simulink model "sing_phase_inv"  (R2020b)
settings: Solver=VariableStepAuto  StartTime=0.0  StopTime=0.3  RelTol=1e-3
libraries: spsMosfetLib x4, spsCurrentMeasurementLib x2, simulink x1, spsDCVoltageSourceLib x1, spsSeriesRLCBranchLib x1, spsVoltageMeasurementLib x1, spspowerguiLib x1
settings Model: Creator=win10  LastModifiedBy=mansi
settings DataIOCC: ReturnWorkspaceOutputs=off

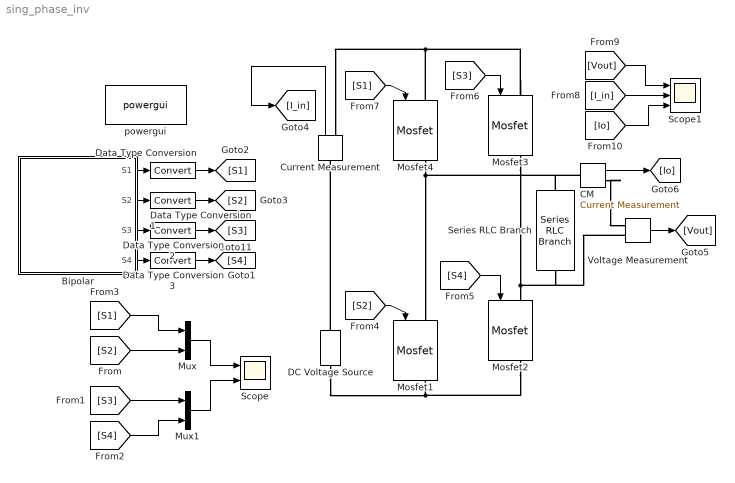
== system sing_phase_inv ==
  Bipolar : Subsystem
  CM : spsCurrentMeasurementLib/Current Measurement  PhasorSimulation=off  OutputType=Complex  PSBequivalent=0
  Current Measurement : spsCurrentMeasurementLib/Current Measurement  PhasorSimulation=off  OutputType=Complex  PSBequivalent=0
  DC Voltage Source : spsDCVoltageSourceLib/DC Voltage Source  Amplitude=400  Measurements=None
  Data Type Conversion{,1..3} (4 alike) : DataTypeConversion
  Mosfet{1..4} (4 alike) : spsMosfetLib/Mosfet  Ron=20e-3  Lon=0  Rd=1e-3  Vfd=0.7  IC=0  Rs=1e5  Cs=inf  Measurements=on
  Mux : Mux  Inputs=2
  Mux1 : Mux  Inputs=2
  Scope : Scope  NumInputPorts=2
  Scope1 : Scope  NumInputPorts=3
  Series RLC Branch : spsSeriesRLCBranchLib/Series RLC Branch  LConnTagsString=__new0  RConnTagsString=__new0  BranchType=R  Resistance=40  Inductance=1e-3  SetiL0=off  InitialCurrent=0  Capacitance=1e-6  Setx0=off  InitialVoltage=0  Measurements=None
  Voltage Measurement : spsVoltageMeasurementLib/Voltage Measurement  PhasorSimulation=off  OutputType=Complex  PSBequivalent=0
  powergui : spspowerguiLib/powergui  Priority=1  SimulationMode=Discrete  SampleTime=1e-7  frequency=60  Iterations=50  frequencyindice=0  Pbase=100e6  ErrMax=1e-4  UnitsV=kV  UnitsW=MW  buscounter=0  FunctionMessages=off  echomessages=off  EnableUseOfTLC=off  CurrentSourceSwitches=off  DisableSnubberDevices=off  DisableRonSwitches=off  DisableVfSwitches=off  DisplayEquations=off  AutomaticDiscreteSolvers=off  SolverType=Tustin/Backward Euler (TBE)  Interpol=off  ExternalGateDelay=off  methode=off  Ts=100  x0status=blocks  SPID=on  SwTol=0  HookPort=off  NonlinearTolerance=1e-4  nMaxIteration=100  ContinueOnMaxIteration=off  RestoreLinks=warning  ResistiveCurrentMeasurement=off  Frange=[0:2:500]  Ylog=off  Xlog=on  ShowGrid=off  save=off  variable=ZData  structure=vo  ZoomFFT=off  StartTime=0.0  cycles=10  DisplayStyle=1  fundamental=50  FreqAxis=off  MaxFrequency=1000  frequencyindicesteady=1  RmsSteady=1  display=off
  wires:
  [S1] -> Mux/1
  [S2] -> Mux/2
  [S3] -> Mux1/1
  [S4] -> Mux1/2
  Mux/1 -> Scope/1
  Mux1/1 -> Scope/2
  [S1] -> Mosfet4/1
  [S3] -> Mosfet3/1
  [S4] -> Mosfet2/1
  [S2] -> Mosfet1/1
  Current Measurement/1 -> [I_in]
  Voltage Measurement/1 -> [Vout]
  [Vout] -> Scope1/1
  [I_in] -> Scope1/2
  CM/1 -> [Io]
  [Io] -> Scope1/3
  Bipolar/3(S3) -> Data Type Conversion2/1
  Data Type Conversion3/1 -> [S4]
  Data Type Conversion/1 -> [S1]
  Data Type Conversion2/1 -> [S3]
  Bipolar/2(S2) -> Data Type Conversion1/1
  Bipolar/4(S4) -> Data Type Conversion3/1
  Bipolar/1(S1) -> Data Type Conversion/1
  Data Type Conversion1/1 -> [S2]
  connections:
  DC Voltage Source/RConn1 -- Current Measurement/LConn1
  DC Voltage Source/LConn1 -- Mosfet2/RConn1 -- Mosfet1/RConn1
  Mosfet3/RConn1 -- Voltage Measurement/LConn2 -- Series RLC Branch/RConn1 -- Mosfet2/LConn1
  Mosfet3/LConn1 -- Current Measurement/RConn1 -- Mosfet4/LConn1
  Mosfet4/RConn1 -- CM/LConn1 -- Series RLC Branch/LConn1 -- Mosfet1/LConn1
  CM/RConn1 -- Voltage Measurement/LConn1

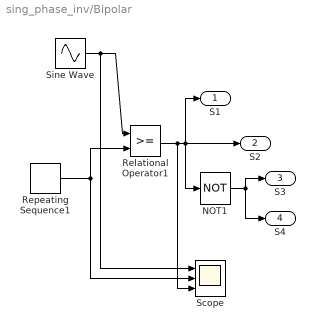
== system sing_phase_inv/Bipolar ==
  NOT1 : Logic  Operator=NOT  AllPortsSameDT=off  OutDataTypeStr=boolean
  Relational Operator1 : RelationalOperator  OutDataTypeStr=boolean  RndMeth=Nearest
  Repeating Sequence1 : simulink/Sources/Repeating Sequence  rep_seq_t=[0 0.00001 0.00002 0.00003 0.00004]  rep_seq_y=[0 1 0 -1 0]
  Scope : Scope  NumInputPorts=3
  Sine Wave : Sin  Amplitude=.95  Frequency=2*pi*50  SampleTime=0
  S1 : Outport
  S2 : Outport  Port=2
  S3 : Outport  Port=3
  S4 : Outport  Port=4
  wires:
  Sine Wave/1 -> Scope/1, Relational Operator1/1
  Relational Operator1/1 -> Scope/3, S1/1, S2/1, NOT1/1
  NOT1/1 -> S3/1, S4/1
  Repeating Sequence1/1 -> Relational Operator1/2, Scope/2
